simulink model "sim_1"  (R2022b)
settings: Solver=FixedStepAuto  StartTime=0.0  StopTime=50  FixedStep=1  RelTol=1e-3
values from neighbouring files (symbols this model uses):
  Wd = c2d(W, T0)    [task_1.m]
settings Model: Creator=mrxmi  LastModifiedBy=mrxmi

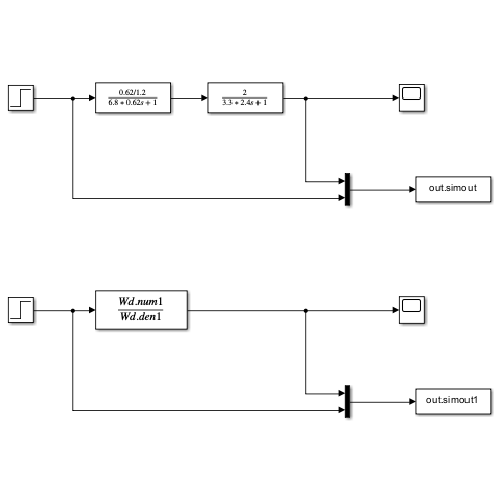
[thumbnail: Simulink's stored preview of the top-level diagram]
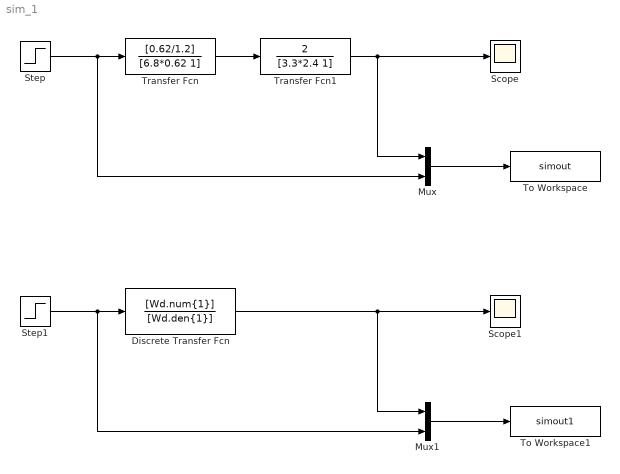
== system sim_1 ==
  Discrete Transfer Fcn : DiscreteTransferFcn  Numerator=[Wd.num{1}]  Denominator=[Wd.den{1}]
  Mux : Mux  Inputs=2
  Mux1 : Mux  Inputs=2
  Scope : Scope
  Scope1 : Scope
  Step : Step  SampleTime=0
  Step1 : Step  Time=0  After=5  SampleTime=0
  To Workspace : ToWorkspace  VariableName=simout  SaveFormat=Structure With Time  SampleTime=-1
  To Workspace1 : ToWorkspace  VariableName=simout1  SaveFormat=Structure With Time  SampleTime=-1
  Transfer Fcn : TransferFcn  Numerator=[0.62/1.2]  Denominator=[6.8*0.62 1]
  Transfer Fcn1 : TransferFcn  Numerator=[2]  Denominator=[3.3*2.4 1]
  wires:
  Transfer Fcn/1 -> Transfer Fcn1/1
  Transfer Fcn1/1 -> Mux/1, Scope/1
  Step/1 -> Transfer Fcn/1, Mux/2
  Mux/1 -> To Workspace/1
  Discrete Transfer Fcn/1 -> Mux1/1, Scope1/1
  Step1/1 -> Discrete Transfer Fcn/1, Mux1/2
  Mux1/1 -> To Workspace1/1
